simulink model "V2GSimulation15"  (R2017b)
settings: Solver=VariableStepAuto  StartTime=0.0  StopTime=inf  MaxStep=1e-4  RelTol=1e-3  EnableMultiTasking=on
undefined symbols (not defined in the file): Ion, Lithium
libraries: powerlib x47, simulink x9, powerlib_meascontrol x9, electricdrivelib x1
settings Model: Creator=Nadir  LastModifiedBy=Korisnik
settings DataIOCC: ReturnWorkspaceOutputs=on
settings OptimizationCC: BlockReduction=off  LifeSpan=inf
settings DebuggingCC: UnconnectedInputMsg=none  UnconnectedOutputMsg=none  UnconnectedLineMsg=none  SFExecutionAtInitializationDiag=none
settings ModelReferenceCC: EnableRefExpFcnMdlSchedulingChecks=off
settings SFSimCC: SimUseLocalCustomCode=on
settings RTWCC: Description=Generic Real-Time Target  RTWUseLocalCustomCode=on
settings CodeAppCC: StateflowObjectComments=on
settings ConfigComp: CovHtmlReporting=on
settings SimscapeCC: SimscapeNormalizeSystem=off

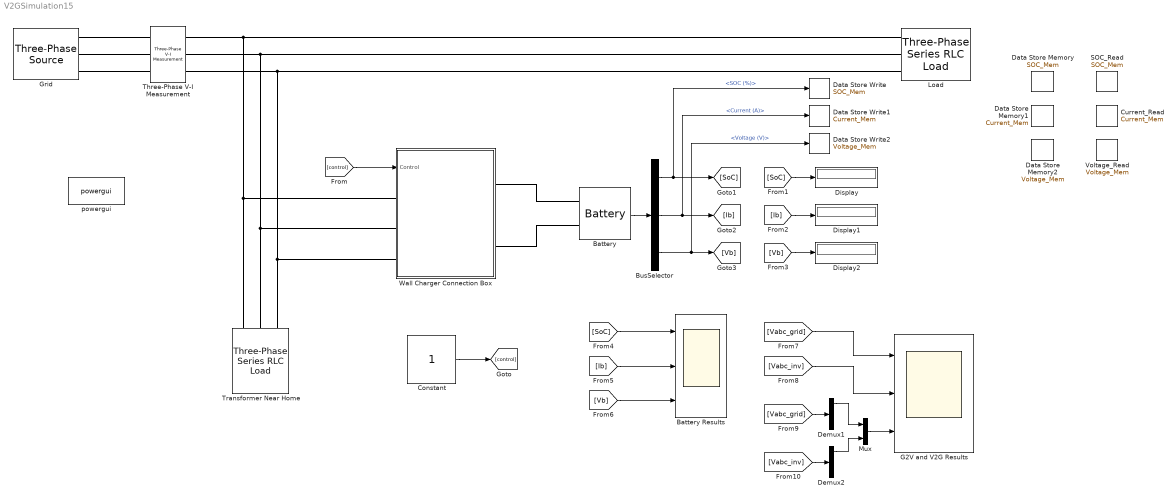
== system V2GSimulation15 ==
  Battery : electricdrivelib/Extra Sources/Battery  BatType=Lithium-Ion  ShowTempParam=off  ThermalPreset=no  ShowAgeParam=off  NomV=230  NomQ=100  SOC=60  Batt_Tr=1e-3  PresetModel=on  MaxQ=100  MinV=172.5  FullV=267.717  Dis_rate=43.4783  R=0.023  Normal_OP=90.4348  expZone="[248.4887      4.913043]"  current=[6.5 13 32.5]  Units=Time  Tci=20  NomT=20  T2=-30  MaxQ2=4.8  FullV2=7.1  Normal_OP2=5.72  expZone2="[6.58  1]"  Rca=0.6  ti=1000  Dp=0  Neq0=0  Tsim=1e6  Ta1=25  Qeol=5.4*0.9  Reol=0.013333*1.2  Char_age=[2.3478, 3]  Dis_age=[2.3478, 10]  N1=1500  N2=10500  N3=1000  N4=1400  Ta2=45  N5=950
  Battery Results : Scope  NumInputPorts=3
  BusSelector : BusSelector  OutputSignals=SOC (%),Current (A),Voltage (V)
  Constant : Constant  OutDataTypeStr=boolean
  Current_Read : DataStoreRead  DataStoreName=Current_Mem
  Data Store Memory : DataStoreMemory  DataStoreName=SOC_Mem  ReadBeforeWriteMsg=warning  WriteAfterWriteMsg=warning  WriteAfterReadMsg=warning  ShowAdditionalParam=off
  Data Store Memory1 : DataStoreMemory  DataStoreName=Current_Mem  ReadBeforeWriteMsg=warning  WriteAfterWriteMsg=warning  WriteAfterReadMsg=warning  ShowAdditionalParam=off
  Data Store Memory2 : DataStoreMemory  DataStoreName=Voltage_Mem  ReadBeforeWriteMsg=warning  WriteAfterWriteMsg=warning  WriteAfterReadMsg=warning  ShowAdditionalParam=off
  Data Store Write : DataStoreWrite  DataStoreName=SOC_Mem
  Data Store Write1 : DataStoreWrite  DataStoreName=Current_Mem
  Data Store Write2 : DataStoreWrite  DataStoreName=Voltage_Mem
  Demux1 : Demux  Outputs=3
  Demux2 : Demux  Outputs=3
  Display : Display
  Display1 : Display
  Display2 : Display
  G2V and V2G Results : Scope  NumInputPorts=3
  Grid : powerlib/Electrical Sources/Three-Phase Source  InternalConnection=Yg  VoltagePhases=off  Voltage=380  PhaseAngle=0  Voltage_phases=[25e3 25e3 25e3]/sqrt(3)  PhaseAngles_phases=[0 -120 +120]  Frequency=50  NonIdealSource=on  SpecifyImpedance=on  Resistance=0.8929  Inductance=16.58e-3  ShortCircuitLevel=100e6  BaseVoltage=380  XRratio=7  BusType=swing  Pref=10e3  Qref=0  Prefabc=[10e3, 10e3, 10e3]  Qrefabc=[0, 0, 0]  Qmin=-inf  Qmax=inf
  Load : powerlib/Elements/Three-Phase Series RLC Load  LConnTagsString=A|B|C  Configuration=Y (grounded)  NominalVoltage=380  Vabc=[1e3 1e3 1e3]  Vabcp=[1e3 1e3 1e3]  NominalFrequency=50  UnbalancedPower=off  ActivePower=10e3  InductivePower=0  CapacitivePower=0  Pabc=[10e3 9e3 11e3]  QLabc=[100 90 110]  QCabc=[100 90 110]  Pabcp=[10e3 9e3 11e3]  QLabcp=[100 90 110]  QCabcp=[100 90 110]  Measurements=None  LoadType=constant Z
  Mux : Mux  Inputs=2
  SOC_Read : DataStoreRead  DataStoreName=SOC_Mem
  Three-Phase V-I Measurement : powerlib/Measurements/Three-Phase V-I Measurement  VoltageMeasurement=phase-to-phase  SetLabelV=on  LabelV=Vabc_grid  Vpu=off  VpuLL=off  CurrentMeasurement=yes  SetLabelI=on  LabelI=Iabc_grid  Ipu=off  Pbase=100e6  Vbase=500e3  OutputType=Complex  PhasorSimulation=off  PSBequivalent=0
  Transformer Near Home : powerlib/Elements/Three-Phase Series RLC Load  LConnTagsString=A|B|C  Configuration=Y (grounded)  NominalVoltage=380  Vabc=[1e3 1e3 1e3]  Vabcp=[1e3 1e3 1e3]  NominalFrequency=50  UnbalancedPower=off  ActivePower=10e3  InductivePower=0  CapacitivePower=0  Pabc=[10e3 9e3 11e3]  QLabc=[100 90 110]  QCabc=[100 90 110]  Pabcp=[10e3 9e3 11e3]  QLabcp=[100 90 110]  QCabcp=[100 90 110]  Measurements=None  LoadType=constant Z
  Voltage_Read : DataStoreRead  DataStoreName=Voltage_Mem
  Wall Charger Connection Box : Subsystem
  powergui : powerlib/powergui  Priority=1  SimulationMode=Continuous  SampleTime=5e-6  frequency=60  Iterations=50  frequencyindice=50  Pbase=100e6  ErrMax=1e-4  UnitsV=kV  UnitsW=MW  buscounter=0  FunctionMessages=off  echomessages=off  EnableUseOfTLC=off  CurrentSourceSwitches=off  DisableSnubberDevices=off  DisableRonSwitches=off  DisableVfSwitches=off  DisplayEquations=off  SolverType=Tustin/Backward Euler (TBE)  Interpol=off  ExternalGateDelay=off  methode=off  Ts=100  x0status=blocks  SPID=on  SwTol=0  HookPort=off  RestoreLinks=warning  ResistiveCurrentMeasurement=off  Frange=[0:2:500]  Ylog=off  Xlog=on  ShowGrid=off  save=off  variable=ZData  structure=0  ZoomFFT=off  StartTime=0.0  cycles=1  DisplayStyle=1  fundamental=60  FreqAxis=off  MaxFrequency=1000  frequencyindicesteady=1  RmsSteady=1  display=off
  wires:
  [control] -> Wall Charger Connection Box/1(Control)
  Constant/1 -> [control]
  Battery/1 -> BusSelector/1
  BusSelector/1 -> Data Store Write/1, [SoC]  "<SOC (%)>"
  [SoC] -> Display/1
  [Ib] -> Display1/1
  [Vb] -> Display2/1
  [SoC] -> Battery Results/1
  [Ib] -> Battery Results/2
  [Vb] -> Battery Results/3
  [Vabc_grid] -> Demux1/1
  [Vabc_inv] -> Demux2/1
  Demux1/1 -> Mux/1
  Demux2/1 -> Mux/2
  Mux/1 -> G2V and V2G Results/3
  [Vabc_inv] -> G2V and V2G Results/2
  [Vabc_grid] -> G2V and V2G Results/1
  BusSelector/2 -> Data Store Write1/1, [Ib]  "<Current (A)>"
  BusSelector/3 -> Data Store Write2/1, [Vb]  "<Voltage (V)>"
  connections:
  Three-Phase V-I Measurement/RConn1 -- Wall Charger Connection Box/LConn1 -- Transformer Near Home/LConn1 -- Load/LConn1
  Wall Charger Connection Box/LConn2 -- Transformer Near Home/LConn2 -- Three-Phase V-I Measurement/RConn2 -- Load/LConn2
  Wall Charger Connection Box/LConn3 -- Transformer Near Home/LConn3 -- Three-Phase V-I Measurement/RConn3 -- Load/LConn3
  Wall Charger Connection Box/RConn1 -- Battery/LConn1
  Wall Charger Connection Box/RConn2 -- Battery/LConn2
  Three-Phase V-I Measurement/LConn1 -- Grid/RConn1
  Three-Phase V-I Measurement/LConn2 -- Grid/RConn2
  Three-Phase V-I Measurement/LConn3 -- Grid/RConn3

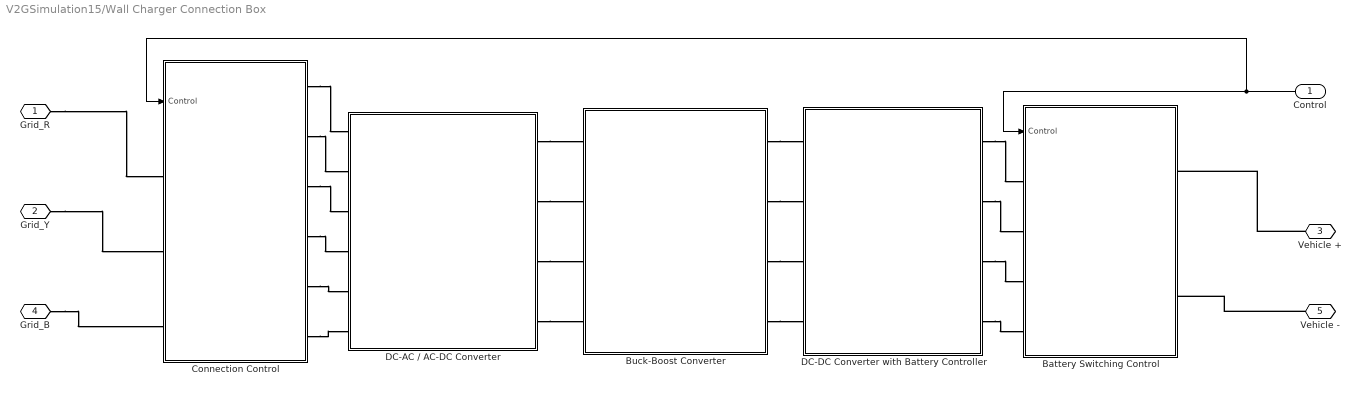
== system V2GSimulation15/Wall Charger Connection Box ==
  Control : Inport
  Battery Switching Control : Subsystem
  Buck-Boost Converter : Subsystem
  Connection Control : Subsystem
  DC-AC / AC-DC Converter : Subsystem
  DC-DC Converter with Battery Controller : Subsystem
  Grid_R : PMIOPort  Port=1  Side=Left
  Grid_Y : PMIOPort  Port=2  Side=Left
  Vehicle + : PMIOPort  Port=3  Side=Right
  Grid_B : PMIOPort  Port=4  Side=Left
  Vehicle - : PMIOPort  Port=5  Side=Right
  wires:
  Control/1 -> Battery Switching Control/1(Control), Connection Control/1(Control)
  connections:
  Connection Control/RConn2 -- DC-AC / AC-DC Converter/LConn2
  DC-DC Converter with Battery Controller/RConn3 -- Battery Switching Control/LConn3
  DC-AC / AC-DC Converter/RConn3 -- Buck-Boost Converter/LConn3
  DC-DC Converter with Battery Controller/RConn1 -- Battery Switching Control/LConn1
  Buck-Boost Converter/RConn2 -- DC-DC Converter with Battery Controller/LConn2
  Buck-Boost Converter/RConn1 -- DC-DC Converter with Battery Controller/LConn1
  Connection Control/RConn3 -- DC-AC / AC-DC Converter/LConn3
  Vehicle -/RConn1 -- Battery Switching Control/RConn2
  Vehicle +/RConn1 -- Battery Switching Control/RConn1
  Grid_B/RConn1 -- Connection Control/LConn3
  Grid_Y/RConn1 -- Connection Control/LConn2
  DC-DC Converter with Battery Controller/RConn4 -- Battery Switching Control/LConn4
  DC-AC / AC-DC Converter/RConn2 -- Buck-Boost Converter/LConn2
  Buck-Boost Converter/RConn3 -- DC-DC Converter with Battery Controller/LConn3
  DC-AC / AC-DC Converter/RConn1 -- Buck-Boost Converter/LConn1
  Buck-Boost Converter/RConn4 -- DC-DC Converter with Battery Controller/LConn4
  Grid_R/RConn1 -- Connection Control/LConn1
  Connection Control/RConn4 -- DC-AC / AC-DC Converter/LConn4
  Connection Control/RConn6 -- DC-AC / AC-DC Converter/LConn6
  DC-AC / AC-DC Converter/RConn4 -- Buck-Boost Converter/LConn4
  DC-DC Converter with Battery Controller/RConn2 -- Battery Switching Control/LConn2
  Connection Control/RConn5 -- DC-AC / AC-DC Converter/LConn5
  Connection Control/RConn1 -- DC-AC / AC-DC Converter/LConn1

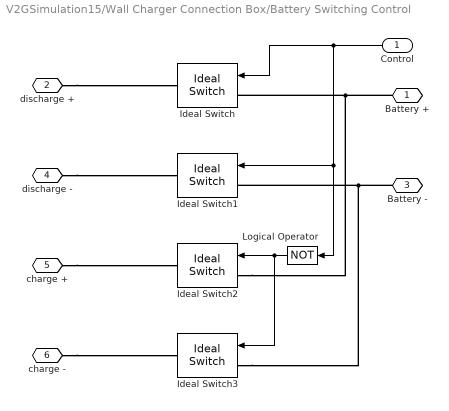
== system V2GSimulation15/Wall Charger Connection Box/Battery Switching Control ==
  Control : Inport
  Ideal Switch{,1..3} (4 alike) : powerlib/Power Electronics/Ideal Switch  Ron=0.001  Lon=0  IC=0  Rs=1e5  Cs=inf  Measurements=off
  Logical Operator : Logic  Operator=NOT  AllPortsSameDT=off  OutDataTypeStr=boolean
  Battery + : PMIOPort  Port=1  Side=Right
  discharge + : PMIOPort  Port=2  Side=Left
  Battery - : PMIOPort  Port=3  Side=Right
  discharge - : PMIOPort  Port=4  Side=Left
  charge + : PMIOPort  Port=5  Side=Left
  charge - : PMIOPort  Port=6  Side=Left
  wires:
  Control/1 -> Ideal Switch1/1, Logical Operator/1, Ideal Switch/1
  Logical Operator/1 -> Ideal Switch3/1, Ideal Switch2/1
  connections:
  charge -/RConn1 -- Ideal Switch3/RConn1
  Ideal Switch3/LConn1 -- Ideal Switch1/LConn1 -- Battery -/RConn1
  Ideal Switch2/LConn1 -- Ideal Switch/LConn1 -- Battery +/RConn1
  discharge +/RConn1 -- Ideal Switch/RConn1
  charge +/RConn1 -- Ideal Switch2/RConn1
  discharge -/RConn1 -- Ideal Switch1/RConn1

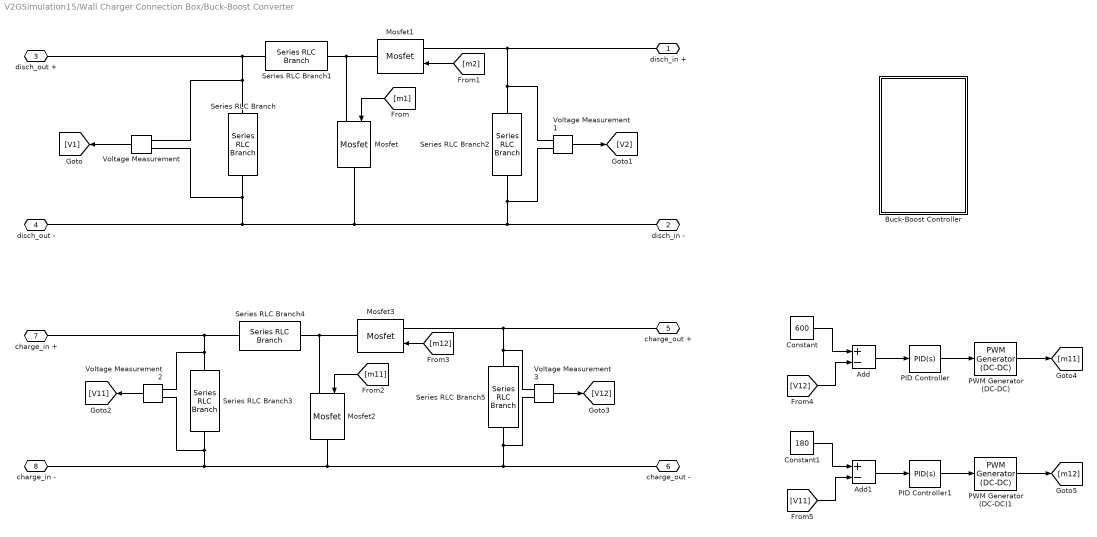
== system V2GSimulation15/Wall Charger Connection Box/Buck-Boost Converter ==
  Add : Sum  Inputs=+-  SaturateOnIntegerOverflow=on  InputSameDT=on  OutDataTypeStr=Inherit: Same as first input
  Add1 : Sum  Inputs=+-  SaturateOnIntegerOverflow=on  InputSameDT=on  OutDataTypeStr=Inherit: Same as first input
  Buck-Boost Controller : Subsystem
  Constant : Constant  Value=600
  Constant1 : Constant  Value=180
  Mosfet{,1..3} (4 alike) : powerlib/Power Electronics/Mosfet  Ron=0.1  Lon=0  Rd=0.01  Vfd=0  IC=0  Rs=1e5  Cs=inf  Measurements=off
  PID Controller : simulink/Continuous/PID Controller  Controller=PID  TimeDomain=Continuous-time  SampleTime=-1  IntegratorMethod=Forward Euler  FilterMethod=Forward Euler  Form=Parallel  UseFilter=on  ControllerParametersSource=internal  P=0  I=7  D=0  N=100  InitialConditionSource=internal  InitialConditionForIntegrator=0  InitialConditionForFilter=0  ExternalReset=none  LimitOutput=off  UpperSaturationLimit=inf  LowerSaturationLimit=-inf  LinearizeAsGain=on  AntiWindupMode=none  Kb=1  TrackingMode=off  Kt=1  PParamMin=[]  PParamMax=[]  IParamMin=[]  IParamMax=[]  DParamMin=[]  DParamMax=[]  NParamMin=[]  NParamMax=[]  KbParamMin=[]  KbParamMax=[]  KtParamMin=[]  KtParamMax=[]  POutMin=[]  POutMax=[]  IOutMin=[]  IOutMax=[]  DOutMin=[]  DOutMax=[]  NOutMin=[]  NOutMax=[]  KbOutMin=[]  KbOutMax=[]  KtOutMin=[]  KtOutMax=[]  IntegratorOutMin=[]  IntegratorOutMax=[]  FilterOutMin=[]  FilterOutMax=[]  SumOutMin=[]  SumOutMax=[]  SumI1OutMin=[]  SumI1OutMax=[]  SumI2OutMin=[]  SumI2OutMax=[]  SumI3OutMin=[]  SumI3OutMax=[]  SumDOutMin=[]  SumDOutMax=[]  SaturationOutMin=[]  SaturationOutMax=[]  IntegratorContinuousStateAttributes=''  IntegratorStateMustResolveToSignalObject=off  IntegratorRTWStateStorageClass=Auto  FilterContinuousStateAttributes=''  FilterStateMustResolveToSignalObject=off  FilterRTWStateStorageClass=Auto  DifferentiatorICPrevScaledInput=0  DifferentiatorOutMin=[]  DifferentiatorOutMax=[]  InitialConditionSetting=State (most efficient)  FilterDiffOutCoefMin=[]  FilterDiffOutCoefMax=[]  SumDenOutMin=[]  SumDenOutMax=[]  SumNumOutMin=[]  SumNumOutMax=[]  ReciprocalOutMin=[]  ReciprocalOutMax=[]  DivideOutMin=[]  DivideOutMax=[]  TunerSelectOption=Transfer Function Based (PID Tuner App)
  PID Controller1 : simulink/Continuous/PID Controller  Controller=PID  TimeDomain=Continuous-time  SampleTime=-1  IntegratorMethod=Forward Euler  FilterMethod=Forward Euler  Form=Parallel  UseFilter=on  ControllerParametersSource=internal  P=0  I=7  D=0  N=100  InitialConditionSource=internal  InitialConditionForIntegrator=0  InitialConditionForFilter=0  ExternalReset=none  LimitOutput=off  UpperSaturationLimit=inf  LowerSaturationLimit=-inf  LinearizeAsGain=on  AntiWindupMode=none  Kb=1  TrackingMode=off  Kt=1  PParamMin=[]  PParamMax=[]  IParamMin=[]  IParamMax=[]  DParamMin=[]  DParamMax=[]  NParamMin=[]  NParamMax=[]  KbParamMin=[]  KbParamMax=[]  KtParamMin=[]  KtParamMax=[]  POutMin=[]  POutMax=[]  IOutMin=[]  IOutMax=[]  DOutMin=[]  DOutMax=[]  NOutMin=[]  NOutMax=[]  KbOutMin=[]  KbOutMax=[]  KtOutMin=[]  KtOutMax=[]  IntegratorOutMin=[]  IntegratorOutMax=[]  FilterOutMin=[]  FilterOutMax=[]  SumOutMin=[]  SumOutMax=[]  SumI1OutMin=[]  SumI1OutMax=[]  SumI2OutMin=[]  SumI2OutMax=[]  SumI3OutMin=[]  SumI3OutMax=[]  SumDOutMin=[]  SumDOutMax=[]  SaturationOutMin=[]  SaturationOutMax=[]  IntegratorContinuousStateAttributes=''  IntegratorStateMustResolveToSignalObject=off  IntegratorRTWStateStorageClass=Auto  FilterContinuousStateAttributes=''  FilterStateMustResolveToSignalObject=off  FilterRTWStateStorageClass=Auto  DifferentiatorICPrevScaledInput=0  DifferentiatorOutMin=[]  DifferentiatorOutMax=[]  InitialConditionSetting=State (most efficient)  FilterDiffOutCoefMin=[]  FilterDiffOutCoefMax=[]  SumDenOutMin=[]  SumDenOutMax=[]  SumNumOutMin=[]  SumNumOutMax=[]  ReciprocalOutMin=[]  ReciprocalOutMax=[]  DivideOutMin=[]  DivideOutMax=[]  TunerSelectOption=Transfer Function Based (PID Tuner App)
  PWM Generator (DC-DC) : powerlib_meascontrol/Pulse & Signal Generators/PWM Generator (DC-DC)  Fsw=5000  Ts=0
  PWM Generator (DC-DC)1 : powerlib_meascontrol/Pulse & Signal Generators/PWM Generator (DC-DC)  Fsw=5000  Ts=0
  Series RLC Branch{,2..3,5} (4 alike) : powerlib/Elements/Series RLC Branch  LConnTagsString=__new0  RConnTagsString=__new0  BranchType=RC  Resistance=0.0001  Inductance=1e-3  SetiL0=off  InitialCurrent=0  Capacitance=1000e-6  Setx0=off  InitialVoltage=0  Measurements=None
  Series RLC Branch1 : powerlib/Elements/Series RLC Branch  LConnTagsString=__new0  RConnTagsString=__new0  BranchType=L  Resistance=1  Inductance=1e-3  SetiL0=off  InitialCurrent=0  Capacitance=1e-6  Setx0=off  InitialVoltage=0  Measurements=None
  Series RLC Branch4 : powerlib/Elements/Series RLC Branch  LConnTagsString=__new0  RConnTagsString=__new0  BranchType=L  Resistance=1  Inductance=1e-3  SetiL0=off  InitialCurrent=0  Capacitance=1e-6  Setx0=off  InitialVoltage=0  Measurements=None
  Voltage Measurement{,1..3} (4 alike) : powerlib/Measurements/Voltage Measurement  PhasorSimulation=off  OutputType=Complex  PSBequivalent=0
  disch_in + : PMIOPort  Port=1  Side=Right
  disch_in - : PMIOPort  Port=2  Side=Right
  disch_out + : PMIOPort  Port=3  Side=Left
  disch_out - : PMIOPort  Port=4  Side=Left
  charge_out + : PMIOPort  Port=5  Side=Right
  charge_out - : PMIOPort  Port=6  Side=Right
  charge_in + : PMIOPort  Port=7  Side=Left
  charge_in - : PMIOPort  Port=8  Side=Left
  wires:
  Add1/1 -> PID Controller1/1
  [m12] -> Mosfet3/1
  PWM Generator (DC-DC)1/1 -> [m12]
  [m1] -> Mosfet/1
  PWM Generator (DC-DC)/1 -> [m11]
  Voltage Measurement1/1 -> [V2]
  Constant/1 -> Add/1
  Voltage Measurement3/1 -> [V12]
  [V11] -> Add1/2
  Add/1 -> PID Controller/1
  Voltage Measurement/1 -> [V1]
  PID Controller1/1 -> PWM Generator (DC-DC)1/1
  PID Controller/1 -> PWM Generator (DC-DC)/1
  Voltage Measurement2/1 -> [V11]
  [V12] -> Add/2
  Constant1/1 -> Add1/1
  [m2] -> Mosfet1/1
  [m11] -> Mosfet2/1
  connections:
  Mosfet3/RConn1 -- Mosfet2/LConn1 -- Series RLC Branch4/LConn1
  Mosfet3/LConn1 -- Voltage Measurement3/LConn1 -- Series RLC Branch5/LConn1 -- charge_out +/RConn1
  Series RLC Branch/RConn1 -- Voltage Measurement/LConn2 -- disch_in -/RConn1 -- Voltage Measurement1/LConn2 -- Series RLC Branch2/RConn1 -- Mosfet/RConn1 -- disch_out -/RConn1
  Series RLC Branch1/RConn1 -- Series RLC Branch/LConn1 -- Voltage Measurement/LConn1 -- disch_out +/RConn1
  Series RLC Branch3/LConn1 -- Voltage Measurement2/LConn1 -- Series RLC Branch4/RConn1 -- charge_in +/RConn1
  Series RLC Branch3/RConn1 -- Voltage Measurement2/LConn2 -- Mosfet2/RConn1 -- charge_out -/RConn1 -- Voltage Measurement3/LConn2 -- Series RLC Branch5/RConn1 -- charge_in -/RConn1
  Mosfet1/LConn1 -- Voltage Measurement1/LConn1 -- Series RLC Branch2/LConn1 -- disch_in +/RConn1
  Mosfet1/RConn1 -- Mosfet/LConn1 -- Series RLC Branch1/LConn1

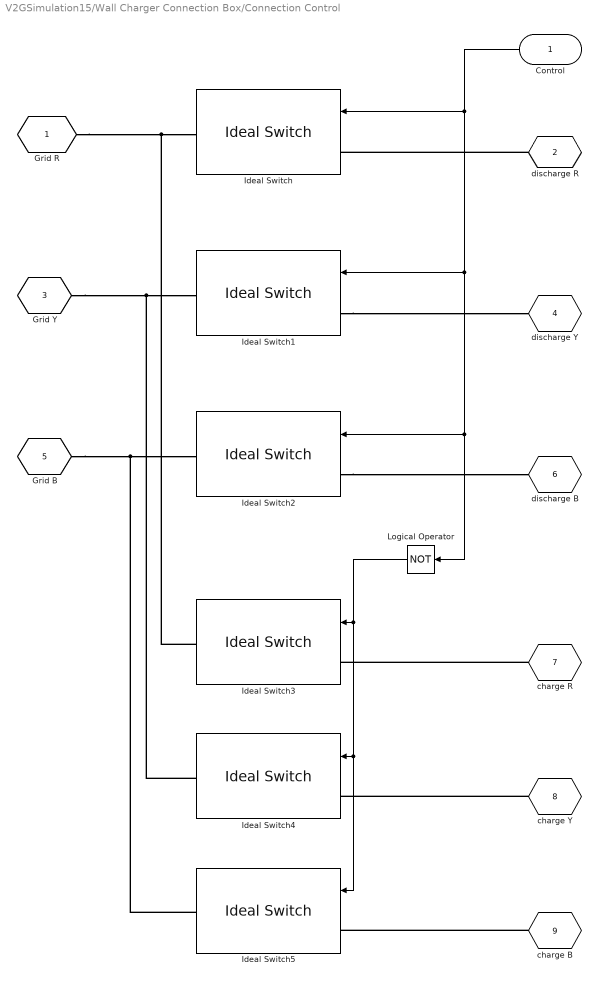
== system V2GSimulation15/Wall Charger Connection Box/Connection Control ==
  Control : Inport
  Ideal Switch{,1..5} (6 alike) : powerlib/Power Electronics/Ideal Switch  Ron=0.001  Lon=0  IC=0  Rs=1e5  Cs=inf  Measurements=off
  Logical Operator : Logic  Operator=NOT  AllPortsSameDT=off  OutDataTypeStr=boolean
  Grid R : PMIOPort  Port=1  Side=Left
  discharge R : PMIOPort  Port=2  Side=Right
  Grid Y : PMIOPort  Port=3  Side=Left
  discharge Y : PMIOPort  Port=4  Side=Right
  Grid B : PMIOPort  Port=5  Side=Left
  discharge B : PMIOPort  Port=6  Side=Right
  charge R : PMIOPort  Port=7  Side=Right
  charge Y : PMIOPort  Port=8  Side=Right
  charge B : PMIOPort  Port=9  Side=Right
  wires:
  Control/1 -> Logical Operator/1, Ideal Switch2/1, Ideal Switch1/1, Ideal Switch/1
  Logical Operator/1 -> Ideal Switch5/1, Ideal Switch4/1, Ideal Switch3/1
  connections:
  Ideal Switch2/LConn1 -- discharge B/RConn1
  Ideal Switch3/RConn1 -- Grid R/RConn1 -- Ideal Switch/RConn1
  charge Y/RConn1 -- Ideal Switch4/LConn1
  Ideal Switch4/RConn1 -- Grid Y/RConn1 -- Ideal Switch1/RConn1
  discharge R/RConn1 -- Ideal Switch/LConn1
  Ideal Switch5/RConn1 -- Grid B/RConn1 -- Ideal Switch2/RConn1
  Ideal Switch1/LConn1 -- discharge Y/RConn1
  charge R/RConn1 -- Ideal Switch3/LConn1
  charge B/RConn1 -- Ideal Switch5/LConn1

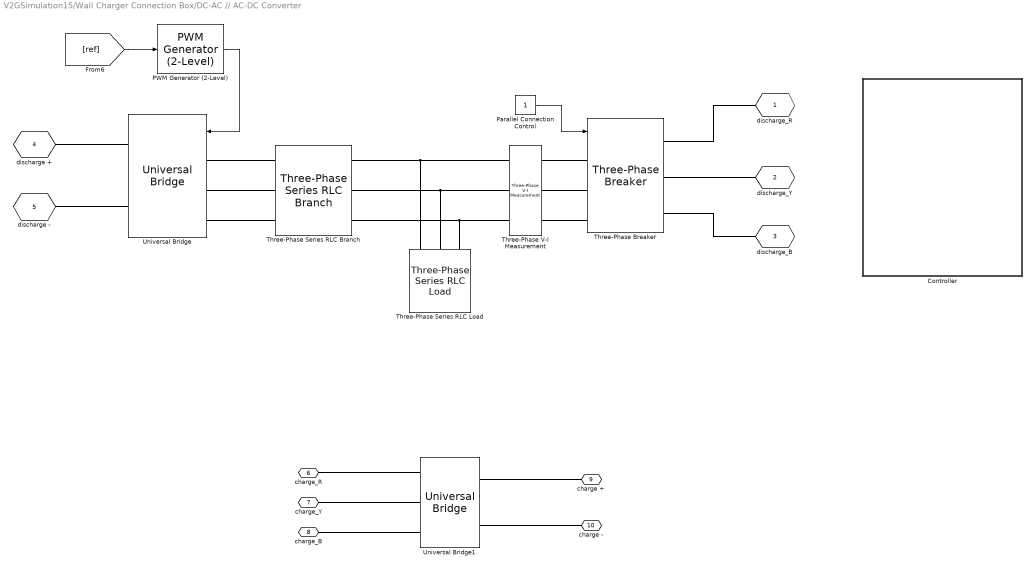
== system V2GSimulation15/Wall Charger Connection Box/DC-AC // AC-DC Converter ==
  Controller : Subsystem
  PWM Generator (2-Level) : powerlib_meascontrol/Pulse & Signal Generators/PWM Generator (2-Level)  ModulatorType=Three-phase bridge (6 pulses)  ModulatorMode=Unsynchronized  Fc=4950  Pc=90  nF=27  MinMax="[ -1  1 ]"  SamplingTechnique=Natural  ModulatingSignals=off  m=0.8  Freq=60  Phase=0  Ts=2.02e-6  ShowCarrierOutport=off
      settings: SourceProductName=Simscape Power Systems
  Parallel Connection Control : Constant  OutDataTypeStr=boolean
  Three-Phase Series RLC Branch : powerlib/Elements/Three-Phase Series RLC Branch  LConnTagsString=A|B|C  RConnTagsString=A|B|C  BranchType=RL  Resistance=0.004332  Inductance=0.0013789184  Capacitance=1e-6  Measurements=None
  Three-Phase Series RLC Load : powerlib/Elements/Three-Phase Series RLC Load  LConnTagsString=A|B|C  Configuration=Delta  NominalVoltage=380  Vabc=[1e3 1e3 1e3]  Vabcp=[1e3 1e3 1e3]  NominalFrequency=50  UnbalancedPower=off  ActivePower=100  InductivePower=0  CapacitivePower=5000  Pabc=[10e3 9e3 11e3]  QLabc=[100 90 110]  QCabc=[100 90 110]  Pabcp=[10e3 9e3 11e3]  QLabcp=[100 90 110]  QCabcp=[100 90 110]  Measurements=None  LoadType=constant Z
  Three-Phase V-I Measurement : powerlib/Measurements/Three-Phase V-I Measurement  VoltageMeasurement=phase-to-phase  SetLabelV=on  LabelV=Vabc_inv  Vpu=off  VpuLL=off  CurrentMeasurement=yes  SetLabelI=on  LabelI=Iabc_inv  Ipu=off  Pbase=100e6  Vbase=500e3  OutputType=Complex  PhasorSimulation=off  PSBequivalent=0
  Three-Phase Breaker : powerlib/Elements/Three-Phase Breaker  InitialState=open  SwitchA=on  SwitchB=on  SwitchC=on  SwitchTimes="[1/60  5/60]"  External=on  BreakerResistance=0.01  SnubberResistance=1e6  SnubberCapacitance=inf  Measurements=None
  Universal Bridge : powerlib/Power Electronics/Universal Bridge  Arms=3  SnubberResistance=1e6  SnubberCapacitance=inf  Device=IGBT / Diodes  Ron=1e-3  Lon=0  ForwardVoltages="[  0  0  ]"  ForwardVoltage=0  GTOparameters=[ 10e-6 , 20e-6 ]  IGBTparameters=[ 1e-6 , 2e-6 ]  Measurements=None  Measurements_2=None  converterType=Rectifier
  Universal Bridge1 : powerlib/Power Electronics/Universal Bridge  Arms=3  SnubberResistance=1e5  SnubberCapacitance=inf  Device=Diodes  Ron=1e-3  Lon=0  ForwardVoltages="[  0  0  ]"  ForwardVoltage=0  GTOparameters=[ 10e-6 , 20e-6 ]  IGBTparameters=[ 1e-6 , 2e-6 ]  Measurements=None  Measurements_2=None  converterType=Rectifier
  discharge_R : PMIOPort  Port=1  Side=Left
  discharge_Y : PMIOPort  Port=2  Side=Left
  discharge_B : PMIOPort  Port=3  Side=Left
  discharge + : PMIOPort  Port=4  Side=Right
  discharge - : PMIOPort  Port=5  Side=Right
  charge_R : PMIOPort  Port=6  Side=Left
  charge_Y : PMIOPort  Port=7  Side=Left
  charge_B : PMIOPort  Port=8  Side=Left
  charge + : PMIOPort  Port=9  Side=Right
  charge - : PMIOPort  Port=10  Side=Right
  wires:
  PWM Generator (2-Level)/1 -> Universal Bridge/1
  [ref] -> PWM Generator (2-Level)/1
  Parallel Connection Control/1 -> Three-Phase Breaker/1
  connections:
  Three-Phase Series RLC Load/LConn1 -- Three-Phase V-I Measurement/LConn1 -- Three-Phase Series RLC Branch/RConn1
  Three-Phase Series RLC Load/LConn2 -- Three-Phase V-I Measurement/LConn2 -- Three-Phase Series RLC Branch/RConn2
  Three-Phase Breaker/RConn2 -- discharge_Y/RConn1
  Three-Phase Breaker/LConn3 -- Three-Phase V-I Measurement/RConn3
  Three-Phase Breaker/RConn3 -- discharge_B/RConn1
  Three-Phase Series RLC Load/LConn3 -- Three-Phase V-I Measurement/LConn3 -- Three-Phase Series RLC Branch/RConn3
  Universal Bridge/RConn1 -- discharge +/RConn1
  charge_B/RConn1 -- Universal Bridge1/LConn3
  Universal Bridge1/RConn2 -- charge -/RConn1
  discharge -/RConn1 -- Universal Bridge/RConn2
  Three-Phase Breaker/RConn1 -- discharge_R/RConn1
  Three-Phase Breaker/LConn2 -- Three-Phase V-I Measurement/RConn2
  Three-Phase Series RLC Branch/LConn2 -- Universal Bridge/LConn2
  charge_Y/RConn1 -- Universal Bridge1/LConn2
  Three-Phase Breaker/LConn1 -- Three-Phase V-I Measurement/RConn1
  Universal Bridge/LConn1 -- Three-Phase Series RLC Branch/LConn1
  Three-Phase Series RLC Branch/LConn3 -- Universal Bridge/LConn3
  Universal Bridge1/RConn1 -- charge +/RConn1
  charge_R/RConn1 -- Universal Bridge1/LConn1

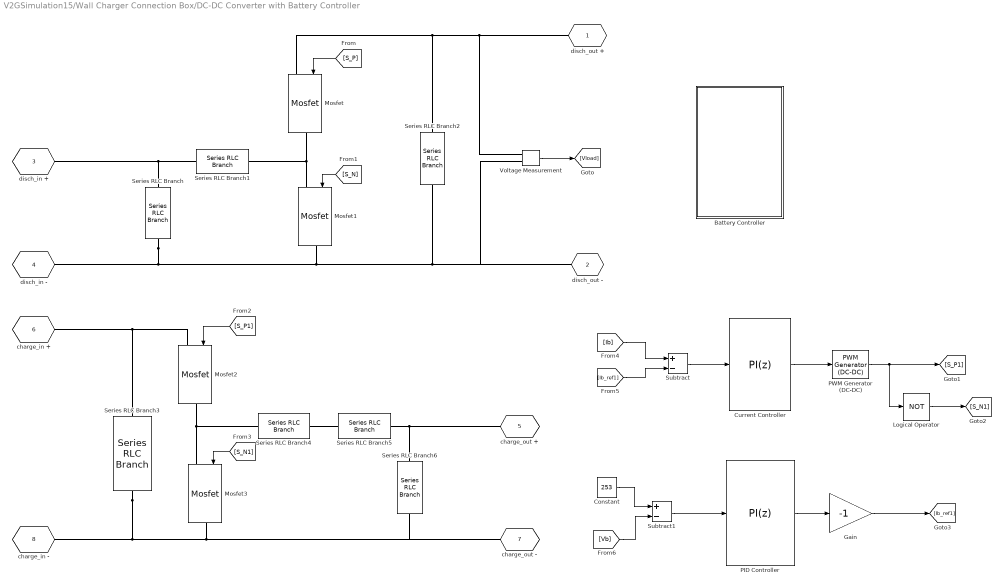
== system V2GSimulation15/Wall Charger Connection Box/DC-DC Converter with Battery Controller ==
  Battery Controller : Subsystem
  Constant : Constant  Value=253
  Current Controller : simulink/Continuous/PID Controller  Controller=PI  TimeDomain=Discrete-time  SampleTime=50e-6  IntegratorMethod=Forward Euler  FilterMethod=Forward Euler  Form=Parallel  UseFilter=on  ControllerParametersSource=internal  P=0.005  I=10  D=0  N=100  InitialConditionSource=internal  InitialConditionForIntegrator=0.54  InitialConditionForFilter=0  ExternalReset=none  LimitOutput=on  UpperSaturationLimit=0.95  LowerSaturationLimit=0  LinearizeAsGain=off  AntiWindupMode=none  Kb=1  TrackingMode=off  Kt=1  PParamMin=[]  PParamMax=[]  IParamMin=[]  IParamMax=[]  DParamMin=[]  DParamMax=[]  NParamMin=[]  NParamMax=[]  KbParamMin=[]  KbParamMax=[]  KtParamMin=[]  KtParamMax=[]  POutMin=[]  POutMax=[]  IOutMin=[]  IOutMax=[]  DOutMin=[]  DOutMax=[]  NOutMin=[]  NOutMax=[]  KbOutMin=[]  KbOutMax=[]  KtOutMin=[]  KtOutMax=[]  IntegratorOutMin=[]  IntegratorOutMax=[]  FilterOutMin=[]  FilterOutMax=[]  SumOutMin=[]  SumOutMax=[]  SumI1OutMin=[]  SumI1OutMax=[]  SumI2OutMin=[]  SumI2OutMax=[]  SumI3OutMin=[]  SumI3OutMax=[]  SumDOutMin=[]  SumDOutMax=[]  SaturationOutMin=[]  SaturationOutMax=[]  IntegratorContinuousStateAttributes=''  IntegratorStateMustResolveToSignalObject=off  IntegratorRTWStateStorageClass=Auto  FilterContinuousStateAttributes=''  FilterStateMustResolveToSignalObject=off  FilterRTWStateStorageClass=Auto  DifferentiatorICPrevScaledInput=0  DifferentiatorOutMin=[]  DifferentiatorOutMax=[]  InitialConditionSetting=State (most efficient)  FilterDiffOutCoefMin=[]  FilterDiffOutCoefMax=[]  SumDenOutMin=[]  SumDenOutMax=[]  SumNumOutMin=[]  SumNumOutMax=[]  ReciprocalOutMin=[]  ReciprocalOutMax=[]  DivideOutMin=[]  DivideOutMax=[]  TunerSelectOption=Transfer Function Based (PID Tuner App)
  Gain : Gain  Gain=-1  SaturateOnIntegerOverflow=on  OutDataTypeStr=Inherit: Same as input  ParamDataTypeStr=Inherit: Same as input
  Logical Operator : Logic  Operator=NOT  AllPortsSameDT=off  OutDataTypeStr=boolean
  Mosfet{,1..3} (4 alike) : powerlib/Power Electronics/Mosfet  Ron=0.1  Lon=0  Rd=0.01  Vfd=0  IC=0  Rs=1e5  Cs=inf  Measurements=off
  PID Controller : simulink/Continuous/PID Controller  Controller=PI  TimeDomain=Discrete-time  SampleTime=50e-6  IntegratorMethod=Forward Euler  FilterMethod=Forward Euler  Form=Parallel  UseFilter=on  ControllerParametersSource=internal  P=40  I=2000  D=0  N=100  InitialConditionSource=internal  InitialConditionForIntegrator=0  InitialConditionForFilter=0  ExternalReset=none  LimitOutput=on  UpperSaturationLimit=22  LowerSaturationLimit=0  LinearizeAsGain=off  AntiWindupMode=none  Kb=1  TrackingMode=off  Kt=1  PParamMin=[]  PParamMax=[]  IParamMin=[]  IParamMax=[]  DParamMin=[]  DParamMax=[]  NParamMin=[]  NParamMax=[]  KbParamMin=[]  KbParamMax=[]  KtParamMin=[]  KtParamMax=[]  POutMin=[]  POutMax=[]  IOutMin=[]  IOutMax=[]  DOutMin=[]  DOutMax=[]  NOutMin=[]  NOutMax=[]  KbOutMin=[]  KbOutMax=[]  KtOutMin=[]  KtOutMax=[]  IntegratorOutMin=[]  IntegratorOutMax=[]  FilterOutMin=[]  FilterOutMax=[]  SumOutMin=[]  SumOutMax=[]  SumI1OutMin=[]  SumI1OutMax=[]  SumI2OutMin=[]  SumI2OutMax=[]  SumI3OutMin=[]  SumI3OutMax=[]  SumDOutMin=[]  SumDOutMax=[]  SaturationOutMin=[]  SaturationOutMax=[]  IntegratorContinuousStateAttributes=''  IntegratorStateMustResolveToSignalObject=off  IntegratorRTWStateStorageClass=Auto  FilterContinuousStateAttributes=''  FilterStateMustResolveToSignalObject=off  FilterRTWStateStorageClass=Auto  DifferentiatorICPrevScaledInput=0  DifferentiatorOutMin=[]  DifferentiatorOutMax=[]  InitialConditionSetting=State (most efficient)  FilterDiffOutCoefMin=[]  FilterDiffOutCoefMax=[]  SumDenOutMin=[]  SumDenOutMax=[]  SumNumOutMin=[]  SumNumOutMax=[]  ReciprocalOutMin=[]  ReciprocalOutMax=[]  DivideOutMin=[]  DivideOutMax=[]  TunerSelectOption=Transfer Function Based (PID Tuner App)
  PWM Generator (DC-DC) : powerlib_meascontrol/Pulse & Signal Generators/PWM Generator (DC-DC)  Fsw=10e3  Ts=5e-6
  Series RLC Branch : powerlib/Elements/Series RLC Branch  LConnTagsString=__new0  RConnTagsString=__new0  BranchType=R  Resistance=10  Inductance=1e-3  SetiL0=off  InitialCurrent=0  Capacitance=1e-6  Setx0=off  InitialVoltage=0  Measurements=None
  Series RLC Branch1 : powerlib/Elements/Series RLC Branch  LConnTagsString=__new0  RConnTagsString=__new0  BranchType=RL  Resistance=0.05  Inductance=5.76e-4  SetiL0=off  InitialCurrent=0  Capacitance=1e-6  Setx0=off  InitialVoltage=0  Measurements=None
  Series RLC Branch2 : powerlib/Elements/Series RLC Branch  LConnTagsString=__new0  RConnTagsString=__new0  BranchType=RC  Resistance=0.001  Inductance=1e-3  SetiL0=off  InitialCurrent=0  Capacitance=1000e-6  Setx0=off  InitialVoltage=0  Measurements=None
  Series RLC Branch3 : powerlib/Elements/Series RLC Branch  LConnTagsString=__new0  RConnTagsString=__new0  BranchType=RC  Resistance=0.001  Inductance=1e-3  SetiL0=off  InitialCurrent=0  Capacitance=1000e-6  Setx0=off  InitialVoltage=0  Measurements=None
  Series RLC Branch4 : powerlib/Elements/Series RLC Branch  LConnTagsString=__new0  RConnTagsString=__new0  BranchType=RL  Resistance=0.05  Inductance=5.76e-4  SetiL0=off  InitialCurrent=0  Capacitance=1e-6  Setx0=off  InitialVoltage=0  Measurements=None
  Series RLC Branch5 : powerlib/Elements/Series RLC Branch  LConnTagsString=__new0  RConnTagsString=__new0  BranchType=R  Resistance=10  Inductance=1e-3  SetiL0=off  InitialCurrent=0  Capacitance=1e-6  Setx0=off  InitialVoltage=0  Measurements=None
  Series RLC Branch6 : powerlib/Elements/Series RLC Branch  LConnTagsString=__new0  RConnTagsString=__new0  BranchType=RC  Resistance=1e-3  Inductance=1e-3  SetiL0=off  InitialCurrent=0  Capacitance=5600e-6  Setx0=off  InitialVoltage=0  Measurements=None
  Subtract : Sum  Inputs=+-  SaturateOnIntegerOverflow=on  InputSameDT=on  OutDataTypeStr=Inherit: Same as first input
  Subtract1 : Sum  Inputs=+-  SaturateOnIntegerOverflow=on  InputSameDT=on  OutDataTypeStr=Inherit: Same as first input
  Voltage Measurement : powerlib/Measurements/Voltage Measurement  PhasorSimulation=off  OutputType=Complex  PSBequivalent=0
  disch_out + : PMIOPort  Port=1  Side=Left
  disch_out - : PMIOPort  Port=2  Side=Left
  disch_in + : PMIOPort  Port=3  Side=Right
  disch_in - : PMIOPort  Port=4  Side=Right
  charge_out + : PMIOPort  Port=5  Side=Right
  charge_in + : PMIOPort  Port=6  Side=Left
  charge_out - : PMIOPort  Port=7  Side=Right
  charge_in - : PMIOPort  Port=8  Side=Left
  wires:
  [S_P] -> Mosfet/1
  [S_N1] -> Mosfet3/1
  PWM Generator (DC-DC)/1 -> Logical Operator/1, [S_P1]
  Subtract/1 -> Current Controller/1
  PID Controller/1 -> Gain/1
  [Ib_ref1] -> Subtract/2
  [S_P1] -> Mosfet2/1
  Gain/1 -> [Ib_ref1]
  Voltage Measurement/1 -> [Vload]
  [Ib] -> Subtract/1
  [S_N] -> Mosfet1/1
  Subtract1/1 -> PID Controller/1
  Current Controller/1 -> PWM Generator (DC-DC)/1
  Constant/1 -> Subtract1/1
  [Vb] -> Subtract1/2
  Logical Operator/1 -> [S_N1]
  connections:
  Series RLC Branch4/LConn1 -- Mosfet2/RConn1 -- Mosfet3/LConn1
  Series RLC Branch3/RConn1 -- Mosfet3/RConn1 -- charge_out -/RConn1 -- Series RLC Branch6/RConn1 -- charge_in -/RConn1
  Series RLC Branch/RConn1 -- disch_out -/RConn1 -- Voltage Measurement/LConn2 -- Series RLC Branch2/RConn1 -- Mosfet1/RConn1 -- disch_in -/RConn1
  Series RLC Branch1/LConn1 -- Series RLC Branch/LConn1 -- disch_in +/RConn1
  Mosfet1/LConn1 -- Mosfet/RConn1 -- Series RLC Branch1/RConn1
  Mosfet/LConn1 -- Series RLC Branch2/LConn1 -- Voltage Measurement/LConn1 -- disch_out +/RConn1
  Mosfet2/LConn1 -- Series RLC Branch3/LConn1 -- charge_in +/RConn1
  charge_out +/RConn1 -- Series RLC Branch5/LConn1 -- Series RLC Branch6/LConn1
  Series RLC Branch4/RConn1 -- Series RLC Branch5/RConn1

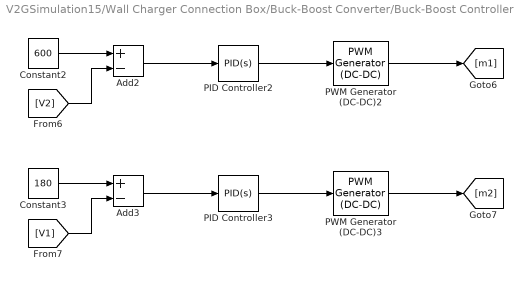
== system V2GSimulation15/Wall Charger Connection Box/Buck-Boost Converter/Buck-Boost Controller ==
  Add2 : Sum  Inputs=+-  SaturateOnIntegerOverflow=on  InputSameDT=on  OutDataTypeStr=Inherit: Same as first input
  Add3 : Sum  Inputs=+-  SaturateOnIntegerOverflow=on  InputSameDT=on  OutDataTypeStr=Inherit: Same as first input
  Constant2 : Constant  Value=600
  Constant3 : Constant  Value=180
  PID Controller2 : simulink/Continuous/PID Controller  Controller=PID  TimeDomain=Continuous-time  SampleTime=-1  IntegratorMethod=Forward Euler  FilterMethod=Forward Euler  Form=Parallel  UseFilter=on  ControllerParametersSource=internal  P=0  I=7  D=0  N=100  InitialConditionSource=internal  InitialConditionForIntegrator=0  InitialConditionForFilter=0  ExternalReset=none  LimitOutput=off  UpperSaturationLimit=inf  LowerSaturationLimit=-inf  LinearizeAsGain=on  AntiWindupMode=none  Kb=1  TrackingMode=off  Kt=1  PParamMin=[]  PParamMax=[]  IParamMin=[]  IParamMax=[]  DParamMin=[]  DParamMax=[]  NParamMin=[]  NParamMax=[]  KbParamMin=[]  KbParamMax=[]  KtParamMin=[]  KtParamMax=[]  POutMin=[]  POutMax=[]  IOutMin=[]  IOutMax=[]  DOutMin=[]  DOutMax=[]  NOutMin=[]  NOutMax=[]  KbOutMin=[]  KbOutMax=[]  KtOutMin=[]  KtOutMax=[]  IntegratorOutMin=[]  IntegratorOutMax=[]  FilterOutMin=[]  FilterOutMax=[]  SumOutMin=[]  SumOutMax=[]  SumI1OutMin=[]  SumI1OutMax=[]  SumI2OutMin=[]  SumI2OutMax=[]  SumI3OutMin=[]  SumI3OutMax=[]  SumDOutMin=[]  SumDOutMax=[]  SaturationOutMin=[]  SaturationOutMax=[]  IntegratorContinuousStateAttributes=''  IntegratorStateMustResolveToSignalObject=off  IntegratorRTWStateStorageClass=Auto  FilterContinuousStateAttributes=''  FilterStateMustResolveToSignalObject=off  FilterRTWStateStorageClass=Auto  DifferentiatorICPrevScaledInput=0  DifferentiatorOutMin=[]  DifferentiatorOutMax=[]  InitialConditionSetting=State (most efficient)  FilterDiffOutCoefMin=[]  FilterDiffOutCoefMax=[]  SumDenOutMin=[]  SumDenOutMax=[]  SumNumOutMin=[]  SumNumOutMax=[]  ReciprocalOutMin=[]  ReciprocalOutMax=[]  DivideOutMin=[]  DivideOutMax=[]  TunerSelectOption=Transfer Function Based (PID Tuner App)
  PID Controller3 : simulink/Continuous/PID Controller  Controller=PID  TimeDomain=Continuous-time  SampleTime=-1  IntegratorMethod=Forward Euler  FilterMethod=Forward Euler  Form=Parallel  UseFilter=on  ControllerParametersSource=internal  P=0  I=7  D=0  N=100  InitialConditionSource=internal  InitialConditionForIntegrator=0  InitialConditionForFilter=0  ExternalReset=none  LimitOutput=off  UpperSaturationLimit=inf  LowerSaturationLimit=-inf  LinearizeAsGain=on  AntiWindupMode=none  Kb=1  TrackingMode=off  Kt=1  PParamMin=[]  PParamMax=[]  IParamMin=[]  IParamMax=[]  DParamMin=[]  DParamMax=[]  NParamMin=[]  NParamMax=[]  KbParamMin=[]  KbParamMax=[]  KtParamMin=[]  KtParamMax=[]  POutMin=[]  POutMax=[]  IOutMin=[]  IOutMax=[]  DOutMin=[]  DOutMax=[]  NOutMin=[]  NOutMax=[]  KbOutMin=[]  KbOutMax=[]  KtOutMin=[]  KtOutMax=[]  IntegratorOutMin=[]  IntegratorOutMax=[]  FilterOutMin=[]  FilterOutMax=[]  SumOutMin=[]  SumOutMax=[]  SumI1OutMin=[]  SumI1OutMax=[]  SumI2OutMin=[]  SumI2OutMax=[]  SumI3OutMin=[]  SumI3OutMax=[]  SumDOutMin=[]  SumDOutMax=[]  SaturationOutMin=[]  SaturationOutMax=[]  IntegratorContinuousStateAttributes=''  IntegratorStateMustResolveToSignalObject=off  IntegratorRTWStateStorageClass=Auto  FilterContinuousStateAttributes=''  FilterStateMustResolveToSignalObject=off  FilterRTWStateStorageClass=Auto  DifferentiatorICPrevScaledInput=0  DifferentiatorOutMin=[]  DifferentiatorOutMax=[]  InitialConditionSetting=State (most efficient)  FilterDiffOutCoefMin=[]  FilterDiffOutCoefMax=[]  SumDenOutMin=[]  SumDenOutMax=[]  SumNumOutMin=[]  SumNumOutMax=[]  ReciprocalOutMin=[]  ReciprocalOutMax=[]  DivideOutMin=[]  DivideOutMax=[]  TunerSelectOption=Transfer Function Based (PID Tuner App)
  PWM Generator (DC-DC)2 : powerlib_meascontrol/Pulse & Signal Generators/PWM Generator (DC-DC)  Fsw=5000  Ts=0
  PWM Generator (DC-DC)3 : powerlib_meascontrol/Pulse & Signal Generators/PWM Generator (DC-DC)  Fsw=5000  Ts=0
  wires:
  PID Controller2/1 -> PWM Generator (DC-DC)2/1
  [V2] -> Add2/2
  [V1] -> Add3/2
  Add3/1 -> PID Controller3/1
  Constant3/1 -> Add3/1
  Add2/1 -> PID Controller2/1
  PWM Generator (DC-DC)2/1 -> [m1]
  PWM Generator (DC-DC)3/1 -> [m2]
  Constant2/1 -> Add2/1
  PID Controller3/1 -> PWM Generator (DC-DC)3/1

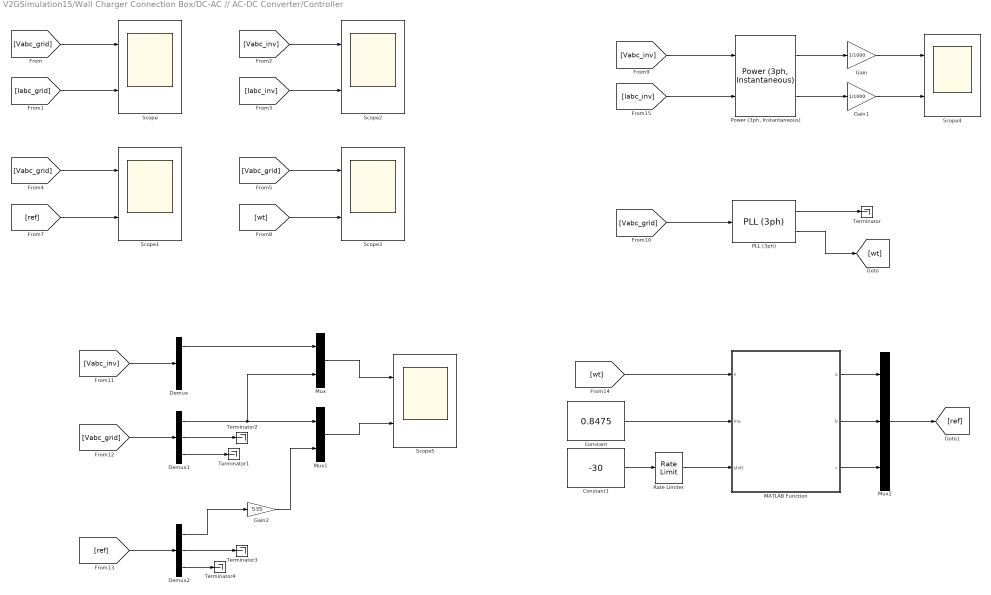
== system V2GSimulation15/Wall Charger Connection Box/DC-AC // AC-DC Converter/Controller ==
  Constant : Constant  Value=0.8475
  Constant1 : Constant  Value=-30
  Demux : Demux  Outputs=3
  Demux1 : Demux  Outputs=3
  Demux2 : Demux  Outputs=3
  Gain : Gain  Gain=1/1000  SaturateOnIntegerOverflow=on  OutDataTypeStr=Inherit: Same as input  ParamDataTypeStr=Inherit: Same as input
  Gain1 : Gain  Gain=1/1000  SaturateOnIntegerOverflow=on  OutDataTypeStr=Inherit: Same as input  ParamDataTypeStr=Inherit: Same as input
  Gain2 : Gain  Gain=535  SaturateOnIntegerOverflow=on  OutDataTypeStr=Inherit: Same as input  ParamDataTypeStr=Inherit: Same as input
  MATLAB Function : MATLAB Function  TreatAsAtomicUnit=on
  Mux : Mux  Inputs=2
  Mux1 : Mux  Inputs=2
  Mux2 : Mux  Inputs=3
  PLL (3ph) : powerlib_meascontrol/PLL/PLL (3ph)  Fmin=45  Par_Init=[0, 50]  ParK=[180, 3200, 1]  TcD=1e-4  MaxRateChangeFreq=12  FilterCutOffFreq=25  Ts=2.02e-6  AGC=on
  "Power (3ph, Instantaneous)" : powerlib_meascontrol/Measurements/Power (3ph, Instantaneous)
      settings: SourceProductName=Simscape Power Systems
  Rate Limiter : RateLimiter
  Scope{,1..5} (6 alike) : Scope  NumInputPorts=2
  Terminator{,1..4} (5 alike) : Terminator
  wires:
  MATLAB Function/3(c) -> Mux2/3
  MATLAB Function/2(b) -> Mux2/2
  Demux1/3 -> Terminator1/1
  Demux2/3 -> Terminator4/1
  Mux/1 -> Scope5/1
  [ref] -> Demux2/1
  [Iabc_grid] -> Scope/2
  Constant/1 -> MATLAB Function/2(ma)
  Demux1/1 -> Mux/2, Mux1/1
  MATLAB Function/1(a) -> Mux2/1
  [Vabc_grid] -> Demux1/1
  Demux2/1 -> Gain2/1
  Constant1/1 -> Rate Limiter/1
  Demux2/2 -> Terminator3/1
  [wt] -> MATLAB Function/1(x)
  Demux/1 -> Mux/1
  Mux1/1 -> Scope5/2
  Demux1/2 -> Terminator2/1
  [Vabc_inv] -> Demux/1
  PLL (3ph)/1 -> Terminator/1
  Rate Limiter/1 -> MATLAB Function/3(shift)
  [Iabc_inv] -> Scope2/2
  [wt] -> Scope3/2
  [Vabc_grid] -> Scope1/1
  [Vabc_grid] -> Scope3/1
  [ref] -> Scope1/2
  [Vabc_grid] -> PLL (3ph)/1
  [Vabc_inv] -> Scope2/1
  Gain/1 -> Scope4/1
  PLL (3ph)/2 -> [wt]
  "Power (3ph, Instantaneous)"/2 -> Gain1/1
  [Vabc_inv] -> "Power (3ph, Instantaneous)"/1
  "Power (3ph, Instantaneous)"/1 -> Gain/1
  [Iabc_inv] -> "Power (3ph, Instantaneous)"/2
  Mux2/1 -> [ref]
  Gain1/1 -> Scope4/2
  [Vabc_grid] -> Scope/1
  Gain2/1 -> Mux1/2

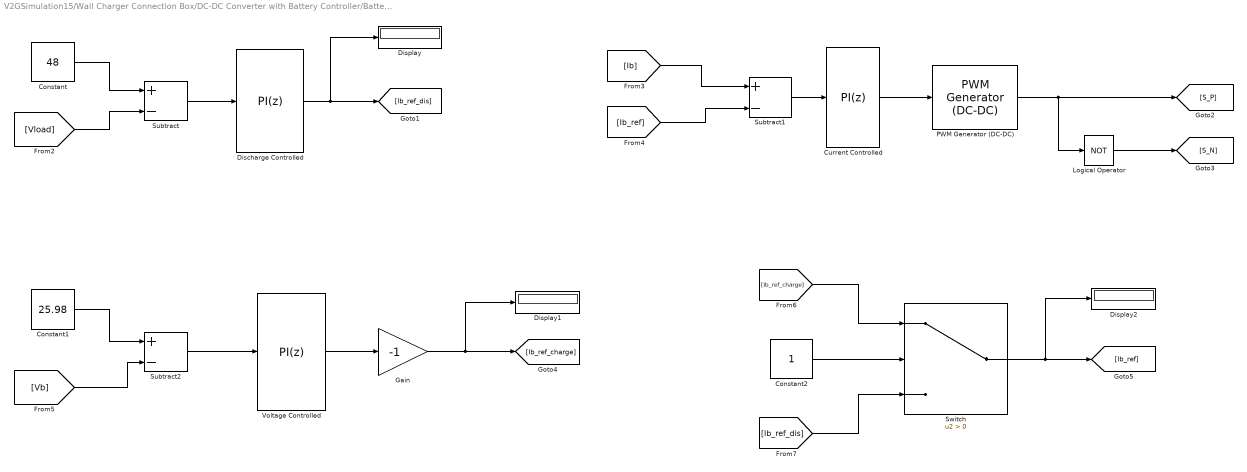
== system V2GSimulation15/Wall Charger Connection Box/DC-DC Converter with Battery Controller/Battery Controller ==
  Constant : Constant  Value=48
  Constant1 : Constant  Value=25.98
  Constant2 : Constant
  Current Controlled : simulink/Continuous/PID Controller  Controller=PI  TimeDomain=Discrete-time  SampleTime=50e-6  IntegratorMethod=Forward Euler  FilterMethod=Forward Euler  Form=Parallel  UseFilter=on  ControllerParametersSource=internal  P=0.005  I=10  D=0  N=100  InitialConditionSource=internal  InitialConditionForIntegrator=0.54  InitialConditionForFilter=0  ExternalReset=none  LimitOutput=on  UpperSaturationLimit=0.95  LowerSaturationLimit=0  LinearizeAsGain=off  AntiWindupMode=none  Kb=1  TrackingMode=off  Kt=1  PParamMin=[]  PParamMax=[]  IParamMin=[]  IParamMax=[]  DParamMin=[]  DParamMax=[]  NParamMin=[]  NParamMax=[]  KbParamMin=[]  KbParamMax=[]  KtParamMin=[]  KtParamMax=[]  POutMin=[]  POutMax=[]  IOutMin=[]  IOutMax=[]  DOutMin=[]  DOutMax=[]  NOutMin=[]  NOutMax=[]  KbOutMin=[]  KbOutMax=[]  KtOutMin=[]  KtOutMax=[]  IntegratorOutMin=[]  IntegratorOutMax=[]  FilterOutMin=[]  FilterOutMax=[]  SumOutMin=[]  SumOutMax=[]  SumI1OutMin=[]  SumI1OutMax=[]  SumI2OutMin=[]  SumI2OutMax=[]  SumI3OutMin=[]  SumI3OutMax=[]  SumDOutMin=[]  SumDOutMax=[]  SaturationOutMin=[]  SaturationOutMax=[]  IntegratorContinuousStateAttributes=''  IntegratorStateMustResolveToSignalObject=off  IntegratorRTWStateStorageClass=Auto  FilterContinuousStateAttributes=''  FilterStateMustResolveToSignalObject=off  FilterRTWStateStorageClass=Auto  DifferentiatorICPrevScaledInput=0  DifferentiatorOutMin=[]  DifferentiatorOutMax=[]  InitialConditionSetting=State (most efficient)  FilterDiffOutCoefMin=[]  FilterDiffOutCoefMax=[]  SumDenOutMin=[]  SumDenOutMax=[]  SumNumOutMin=[]  SumNumOutMax=[]  ReciprocalOutMin=[]  ReciprocalOutMax=[]  DivideOutMin=[]  DivideOutMax=[]  TunerSelectOption=Transfer Function Based (PID Tuner App)
  Discharge Controlled : simulink/Continuous/PID Controller  Controller=PI  TimeDomain=Discrete-time  SampleTime=500e-6  IntegratorMethod=Forward Euler  FilterMethod=Forward Euler  Form=Parallel  UseFilter=on  ControllerParametersSource=internal  P=0.25  I=50  D=0  N=100  InitialConditionSource=internal  InitialConditionForIntegrator=0  InitialConditionForFilter=0  ExternalReset=none  LimitOutput=on  UpperSaturationLimit=22  LowerSaturationLimit=0  LinearizeAsGain=off  AntiWindupMode=none  Kb=1  TrackingMode=off  Kt=1  PParamMin=[]  PParamMax=[]  IParamMin=[]  IParamMax=[]  DParamMin=[]  DParamMax=[]  NParamMin=[]  NParamMax=[]  KbParamMin=[]  KbParamMax=[]  KtParamMin=[]  KtParamMax=[]  POutMin=[]  POutMax=[]  IOutMin=[]  IOutMax=[]  DOutMin=[]  DOutMax=[]  NOutMin=[]  NOutMax=[]  KbOutMin=[]  KbOutMax=[]  KtOutMin=[]  KtOutMax=[]  IntegratorOutMin=[]  IntegratorOutMax=[]  FilterOutMin=[]  FilterOutMax=[]  SumOutMin=[]  SumOutMax=[]  SumI1OutMin=[]  SumI1OutMax=[]  SumI2OutMin=[]  SumI2OutMax=[]  SumI3OutMin=[]  SumI3OutMax=[]  SumDOutMin=[]  SumDOutMax=[]  SaturationOutMin=[]  SaturationOutMax=[]  IntegratorContinuousStateAttributes=''  IntegratorStateMustResolveToSignalObject=off  IntegratorRTWStateStorageClass=Auto  FilterContinuousStateAttributes=''  FilterStateMustResolveToSignalObject=off  FilterRTWStateStorageClass=Auto  DifferentiatorICPrevScaledInput=0  DifferentiatorOutMin=[]  DifferentiatorOutMax=[]  InitialConditionSetting=State (most efficient)  FilterDiffOutCoefMin=[]  FilterDiffOutCoefMax=[]  SumDenOutMin=[]  SumDenOutMax=[]  SumNumOutMin=[]  SumNumOutMax=[]  ReciprocalOutMin=[]  ReciprocalOutMax=[]  DivideOutMin=[]  DivideOutMax=[]  TunerSelectOption=Transfer Function Based (PID Tuner App)
  Display : Display
  Display1 : Display
  Display2 : Display
  Gain : Gain  Gain=-1  SaturateOnIntegerOverflow=on  OutDataTypeStr=Inherit: Same as input  ParamDataTypeStr=Inherit: Same as input
  Logical Operator : Logic  Operator=NOT  AllPortsSameDT=off  OutDataTypeStr=boolean
  PWM Generator (DC-DC) : powerlib_meascontrol/Pulse & Signal Generators/PWM Generator (DC-DC)  Fsw=10e3  Ts=5e-6
  Subtract : Sum  Inputs=+-  SaturateOnIntegerOverflow=on  InputSameDT=on  OutDataTypeStr=Inherit: Same as first input
  Subtract1 : Sum  Inputs=+-  SaturateOnIntegerOverflow=on  InputSameDT=on  OutDataTypeStr=Inherit: Same as first input
  Subtract2 : Sum  Inputs=+-  SaturateOnIntegerOverflow=on  InputSameDT=on  OutDataTypeStr=Inherit: Same as first input
  Switch : Switch  Criteria=u2 > Threshold
  Voltage Controlled : simulink/Continuous/PID Controller  Controller=PI  TimeDomain=Discrete-time  SampleTime=50e-6  IntegratorMethod=Forward Euler  FilterMethod=Forward Euler  Form=Parallel  UseFilter=on  ControllerParametersSource=internal  P=40  I=2000  D=0  N=100  InitialConditionSource=internal  InitialConditionForIntegrator=0  InitialConditionForFilter=0  ExternalReset=none  LimitOutput=on  UpperSaturationLimit=22  LowerSaturationLimit=0  LinearizeAsGain=off  AntiWindupMode=none  Kb=1  TrackingMode=off  Kt=1  PParamMin=[]  PParamMax=[]  IParamMin=[]  IParamMax=[]  DParamMin=[]  DParamMax=[]  NParamMin=[]  NParamMax=[]  KbParamMin=[]  KbParamMax=[]  KtParamMin=[]  KtParamMax=[]  POutMin=[]  POutMax=[]  IOutMin=[]  IOutMax=[]  DOutMin=[]  DOutMax=[]  NOutMin=[]  NOutMax=[]  KbOutMin=[]  KbOutMax=[]  KtOutMin=[]  KtOutMax=[]  IntegratorOutMin=[]  IntegratorOutMax=[]  FilterOutMin=[]  FilterOutMax=[]  SumOutMin=[]  SumOutMax=[]  SumI1OutMin=[]  SumI1OutMax=[]  SumI2OutMin=[]  SumI2OutMax=[]  SumI3OutMin=[]  SumI3OutMax=[]  SumDOutMin=[]  SumDOutMax=[]  SaturationOutMin=[]  SaturationOutMax=[]  IntegratorContinuousStateAttributes=''  IntegratorStateMustResolveToSignalObject=off  IntegratorRTWStateStorageClass=Auto  FilterContinuousStateAttributes=''  FilterStateMustResolveToSignalObject=off  FilterRTWStateStorageClass=Auto  DifferentiatorICPrevScaledInput=0  DifferentiatorOutMin=[]  DifferentiatorOutMax=[]  InitialConditionSetting=State (most efficient)  FilterDiffOutCoefMin=[]  FilterDiffOutCoefMax=[]  SumDenOutMin=[]  SumDenOutMax=[]  SumNumOutMin=[]  SumNumOutMax=[]  ReciprocalOutMin=[]  ReciprocalOutMax=[]  DivideOutMin=[]  DivideOutMax=[]  TunerSelectOption=Transfer Function Based (PID Tuner App)
  wires:
  Switch/1 -> Display2/1, [Ib_ref]
  Current Controlled/1 -> PWM Generator (DC-DC)/1
  Constant2/1 -> Switch/2
  Constant1/1 -> Subtract2/1
  Subtract2/1 -> Voltage Controlled/1
  [Ib_ref_charge] -> Switch/1
  Discharge Controlled/1 -> Display/1, [Ib_ref_dis]
  Logical Operator/1 -> [S_N]
  Voltage Controlled/1 -> Gain/1
  Constant/1 -> Subtract/1
  [Vload] -> Subtract/2
  PWM Generator (DC-DC)/1 -> Logical Operator/1, [S_P]
  [Ib_ref_dis] -> Switch/3
  Gain/1 -> Display1/1, [Ib_ref_charge]
  Subtract/1 -> Discharge Controlled/1
  [Vb] -> Subtract2/2
  [Ib] -> Subtract1/1
  Subtract1/1 -> Current Controlled/1
  [Ib_ref] -> Subtract1/2

== matlab function V2GSimulation15/Wall Charger Connection Box/DC-AC // AC-DC Converter/Controller/MATLAB Function ==
  data: x input; a output; ma input; shift input; b output; c output
function [a, b, c] = ref_generation(x, ma, shift)

shift_k = shift * pi / 180;
a = (ma * (sin((x) + shift_k)));
b = (ma * (sin((x) + shift_k - (2*pi/3))));
c = (ma * (sin((x) + shift_k + (2*pi/3))));
